simulink model "EvReferenceApplication"  (R2018a)
settings: Solver=ode23tb  StartTime=0  StopTime=ttime  RelTol=1e-3  EnableMultiTasking=on
InitFcn:
  | open_system('EvReferenceApplication/Visualization/Performance and FE Scope');
undefined symbols (not defined in the file): const, const1, const2, Grade
libraries: autolibshared x5
settings Model: ModifiedByFormat=The MathWorks, Inc.  SimulationMode=accelerator  PauseTimes=23.46  Creator=The MathWorks, Inc.  LastModifiedBy=The MathWorks, Inc.
settings SolverCC: DecoupledContinuousIntegration=on
settings DataIOCC: DSMLogging=off
settings DebuggingCC: AlgebraicLoopMsg=none  UnderspecifiedInitializationDetection=Classic  MergeDetectMultiDrivingBlocksExec=none  ModelReferenceExtraNoncontSigs=none
settings ModelReferenceCC: UpdateModelReferenceTargets=IfOutOfDate  EnableParallelModelReferenceBuilds=on  ModelReferenceMinAlgLoopOccurrences=on  PropagateSignalLabelsOutOfModel=off
settings CodeAppCC: StateflowObjectComments=on
settings GRTTargetCC: TargetLangStandard=C89/C90 (ANSI)
settings ConfigComp: CovMetricSettings=dsw  CovHtmlReporting=on  CovSaveCumulativeToWorkspaceVar=on  CovSaveSingleToWorkspaceVar=on  CovShowResultsExplorer=off  CovExternalEMLEnable=off

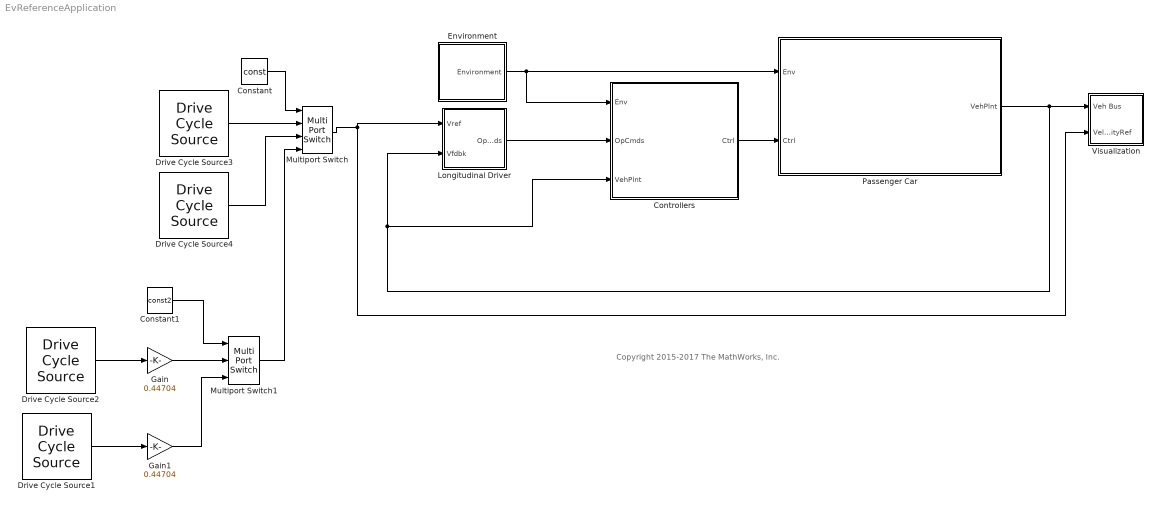
== system EvReferenceApplication ==
  note: Copyright 2015-2017 The MathWorks, Inc.
  Constant : Constant  Value=const
  Constant1 : Constant  Value=const2
  Controllers : Subsystem
      mask Display: image('SystemControllers.png','center')
  Drive Cycle Source1 : autolibshared/Drive Cycle Source  cycleVar=.mat, .xls, .xlsx or .txt file  fileVar=C:\Users\Umar\Software\Matlab\Projects\EV_4\EV\hwfe_1Hz.csv  tfinal="775  seconds"  cycleRepeat=off  outAccPort=off  outGearPort=off  gearList=No gear data  t_wot1=5  xdot_woto=50  xdot_wot1=300  t_wot2=300  xdot_wot2=50  t_wotend=310  srcUnit=mph  outUnit=mph  srcAccUnit=m/s/s  outAccUnit=m/s^2  dt=0  aMode=1
      settings: SourceProductName=Powertrain Blockset  SourceProductBaseCode=PW
  Drive Cycle Source2 : autolibshared/Drive Cycle Source  cycleVar=.mat, .xls, .xlsx or .txt file  fileVar=C:\Users\Umar\Software\Matlab\Projects\EV_4\EV\FTPMC1B.csv  tfinal="1874  seconds"  cycleRepeat=off  outAccPort=off  outGearPort=off  gearList=No gear data  t_wot1=5  xdot_woto=50  xdot_wot1=300  t_wot2=300  xdot_wot2=50  t_wotend=310  srcUnit=mph  outUnit=mph  srcAccUnit=m/s/s  outAccUnit=m/s^2  dt=0  aMode=1
      settings: SourceProductName=Powertrain Blockset  SourceProductBaseCode=PW
  Drive Cycle Source3 : autolibshared/Drive Cycle Source  cycleVar=FTP75  fileVar=L:\Bauto\matlab\test\toolbox\shared\autoblks\scenario\adac.txt  tfinal="2474  seconds"  cycleRepeat=off  outAccPort=off  outGearPort=off  gearList=No gear data  t_wot1=5  xdot_woto=0  xdot_wot1=30  t_wot2=20  xdot_wot2=0  t_wotend=30  srcUnit=m/s  outUnit=m/s  srcAccUnit=m/s/s  outAccUnit=m/s^2  dt=0  aMode=1
      settings: SourceProductName=Powertrain Blockset  SourceProductBaseCode=PW
  Drive Cycle Source4 : autolibshared/Drive Cycle Source  cycleVar=Wide Open Throttle (WOT)  fileVar=L:\Bauto\matlab\test\toolbox\shared\autoblks\scenario\adac.txt  tfinal="310  seconds"  cycleRepeat=off  outAccPort=off  outGearPort=off  gearList=No gear data  t_wot1=5  xdot_woto=0  xdot_wot1=300  t_wot2=300  xdot_wot2=0  t_wotend=310  srcUnit=m/s  outUnit=m/s  srcAccUnit=m/s/s  outAccUnit=m/s^2  dt=0  aMode=1
      settings: SourceProductName=Powertrain Blockset  SourceProductBaseCode=PW
  Environment : Subsystem
      mask Display: disp('Environment')
  Gain : Gain  Gain=0.44704
  Gain1 : Gain  Gain=0.44704
  Longitudinal Driver : Subsystem
      mask Display: image('LongitudinalDriver.png', 'center')
  Multiport Switch : MultiPortSwitch
  Multiport Switch1 : MultiPortSwitch  Inputs=2
  Passenger Car : Subsystem
      mask Display: image('PassengerVehicle.png','center')
  Visualization : Subsystem
      mask Display: disp('Visualization')
  wires:
  Longitudinal Driver/1(OpCmds) -> Controllers/2(OpCmds)
  Environment/1(Environment) -> Controllers/1(Env), Passenger Car/1(Env)
  Controllers/1(Ctrl) -> Passenger Car/2(Ctrl)
  Passenger Car/1(VehPlnt) -> Controllers/3(VehPlnt), Longitudinal Driver/2(Vfdbk), Visualization/1(Veh Bus)
  Multiport Switch/1 -> Longitudinal Driver/1(Vref), Visualization/2(VelocityRef)
  Drive Cycle Source3/1 -> Multiport Switch/2
  Constant/1 -> Multiport Switch/1
  Drive Cycle Source4/1 -> Multiport Switch/3
  Drive Cycle Source2/1 -> Gain/1
  Drive Cycle Source1/1 -> Gain1/1
  Multiport Switch1/1 -> Multiport Switch/4
  Constant1/1 -> Multiport Switch1/1
  Gain/1 -> Multiport Switch1/2
  Gain1/1 -> Multiport Switch1/3

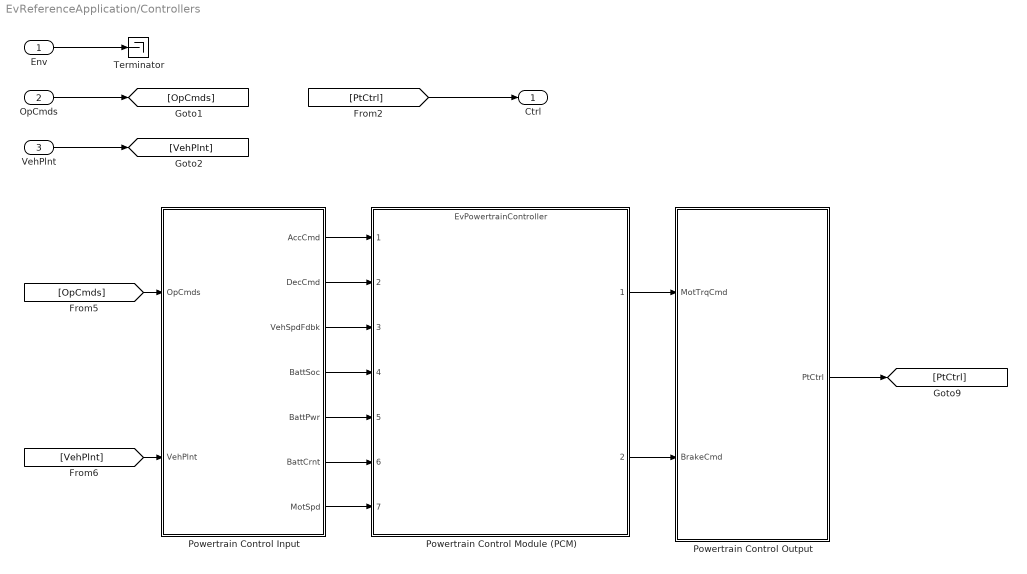
== system EvReferenceApplication/Controllers ==
  Env : Inport
  OpCmds : Inport  Port=2
  VehPlnt : Inport  Port=3
  Powertrain Control Input : Subsystem
  Powertrain Control Module (PCM) : ModelReference  ModelNameDialog=EvPowertrainController  ModelReferenceVersion=1.403
  Powertrain Control Output : Subsystem
  Terminator : Terminator
  Ctrl : Outport
  wires:
  [PtCtrl] -> Ctrl/1
  Env/1 -> Terminator/1
  [OpCmds] -> Powertrain Control Input/1(OpCmds)
  Powertrain Control Output/1(PtCtrl) -> [PtCtrl]
  [VehPlnt] -> Powertrain Control Input/2(VehPlnt)
  VehPlnt/1 -> [VehPlnt]
  OpCmds/1 -> [OpCmds]
  Powertrain Control Input/4(BattSoc) -> Powertrain Control Module (PCM)/4
  Powertrain Control Input/3(VehSpdFdbk) -> Powertrain Control Module (PCM)/3
  Powertrain Control Input/2(DecCmd) -> Powertrain Control Module (PCM)/2
  Powertrain Control Input/1(AccCmd) -> Powertrain Control Module (PCM)/1
  Powertrain Control Input/5(BattPwr) -> Powertrain Control Module (PCM)/5
  Powertrain Control Input/6(BattCrnt) -> Powertrain Control Module (PCM)/6
  Powertrain Control Input/7(MotSpd) -> Powertrain Control Module (PCM)/7
  Powertrain Control Module (PCM)/1 -> Powertrain Control Output/1(MotTrqCmd)
  Powertrain Control Module (PCM)/2 -> Powertrain Control Output/2(BrakeCmd)

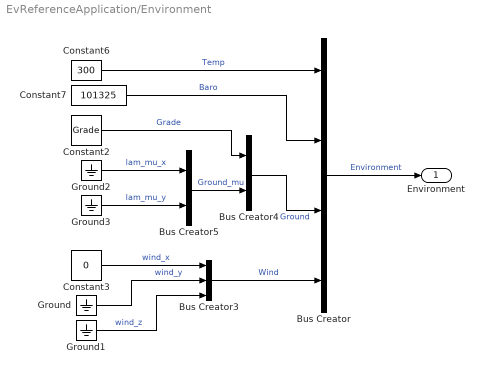
== system EvReferenceApplication/Environment ==
  Bus Creator : BusCreator  Inputs=4
  Bus Creator3 : BusCreator  Inputs=3
  Bus Creator4 : BusCreator  Inputs=2
  Bus Creator5 : BusCreator  Inputs=2
  Constant2 : Constant  Value=Grade
  Constant3 : Constant  Value=0
  Constant6 : Constant  Value=300
  Constant7 : Constant  Value=101325
  Ground{,1..3} (4 alike) : Ground
  Environment : Outport
  wires:
  Ground2/1 -> Bus Creator5/1  "lam_mu_x"
  Ground3/1 -> Bus Creator5/2  "lam_mu_y"
  Bus Creator5/1 -> Bus Creator4/2  "Ground_mu"
  Bus Creator4/1 -> Bus Creator/3  "Ground"
  Bus Creator3/1 -> Bus Creator/4  "Wind"
  Constant3/1 -> Bus Creator3/1  "wind_x"
  Ground/1 -> Bus Creator3/2  "wind_y"
  Ground1/1 -> Bus Creator3/3  "wind_z"
  Constant6/1 -> Bus Creator/1  "Temp"
  Constant2/1 -> Bus Creator4/1  "Grade"
  Bus Creator/1 -> Environment/1  "Environment"
  Constant7/1 -> Bus Creator/2  "Baro"

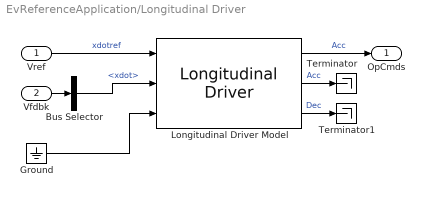
== system EvReferenceApplication/Longitudinal Driver ==
  Vref : Inport
  Vfdbk : Inport  Port=2
  Bus Selector : BusSelector  OutputSignals=Veh.xdot
  Ground : Ground
  Longitudinal Driver Model : autolibshared/Longitudinal Driver  aMode=1  vnom=5  Kp=1.5  Ki=1.5  Kaw=1  Kff=.1  Kg=0  tauerr=0.01
      settings: SourceProductName=Powertrain Blockset  SourceProductBaseCode=PW
  Terminator : Terminator
  Terminator1 : Terminator
  OpCmds : Outport
  wires:
  Bus Selector/1 -> Longitudinal Driver Model/2  "<xdot>"
  Vref/1 -> Longitudinal Driver Model/1  "xdotref"
  Vfdbk/1 -> Bus Selector/1
  Longitudinal Driver Model/1 -> OpCmds/1  "Acc"
  Longitudinal Driver Model/2 -> Terminator/1  "Acc"
  Longitudinal Driver Model/3 -> Terminator1/1  "Dec"
  Ground/1 -> Longitudinal Driver Model/3

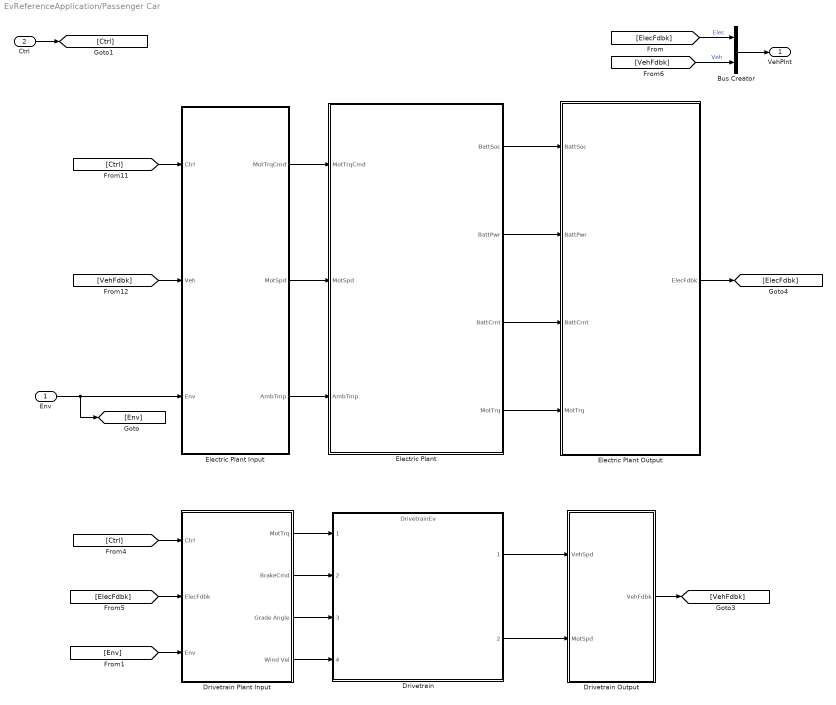
== system EvReferenceApplication/Passenger Car ==
  Env : Inport
  Ctrl : Inport  Port=2
  Bus Creator : BusCreator  Inputs=2
  Drivetrain : ModelReference  ModelNameDialog=DrivetrainEv.slx  SimulationMode=Normal  ModelReferenceVersion=1.431
  Drivetrain Output : Subsystem
  Drivetrain Plant Input : Subsystem
  Electric Plant : Subsystem
  Electric Plant Input : Subsystem
  Electric Plant Output : Subsystem
  VehPlnt : Outport
  wires:
  Ctrl/1 -> [Ctrl]
  Env/1 -> [Env], Electric Plant Input/3(Env)
  [Ctrl] -> Drivetrain Plant Input/1(Ctrl)
  Bus Creator/1 -> VehPlnt/1
  [VehFdbk] -> Bus Creator/2  "Veh"
  Drivetrain Output/1(VehFdbk) -> [VehFdbk]
  Electric Plant Output/1(ElecFdbk) -> [ElecFdbk]
  [ElecFdbk] -> Bus Creator/1  "Elec"
  [Ctrl] -> Electric Plant Input/1(Ctrl)
  [ElecFdbk] -> Drivetrain Plant Input/2(ElecFdbk)
  [VehFdbk] -> Electric Plant Input/2(Veh)
  Drivetrain Plant Input/2(BrakeCmd) -> Drivetrain/2
  Drivetrain Plant Input/1(MotTrq) -> Drivetrain/1
  Drivetrain/2 -> Drivetrain Output/2(MotSpd)
  Drivetrain/1 -> Drivetrain Output/1(VehSpd)
  Electric Plant Input/1(MotTrqCmd) -> Electric Plant/1(MotTrqCmd)
  Electric Plant Input/2(MotSpd) -> Electric Plant/2(MotSpd)
  Electric Plant/1(BattSoc) -> Electric Plant Output/1(BattSoc)
  Electric Plant/2(BattPwr) -> Electric Plant Output/2(BattPwr)
  Electric Plant/3(BattCrnt) -> Electric Plant Output/3(BattCrnt)
  Electric Plant/4(MotTrq) -> Electric Plant Output/4(MotTrq)
  Electric Plant Input/3(AmbTmp) -> Electric Plant/3(AmbTmp)
  [Env] -> Drivetrain Plant Input/3(Env)
  Drivetrain Plant Input/3(Grade Angle) -> Drivetrain/3
  Drivetrain Plant Input/4(Wind Vel) -> Drivetrain/4

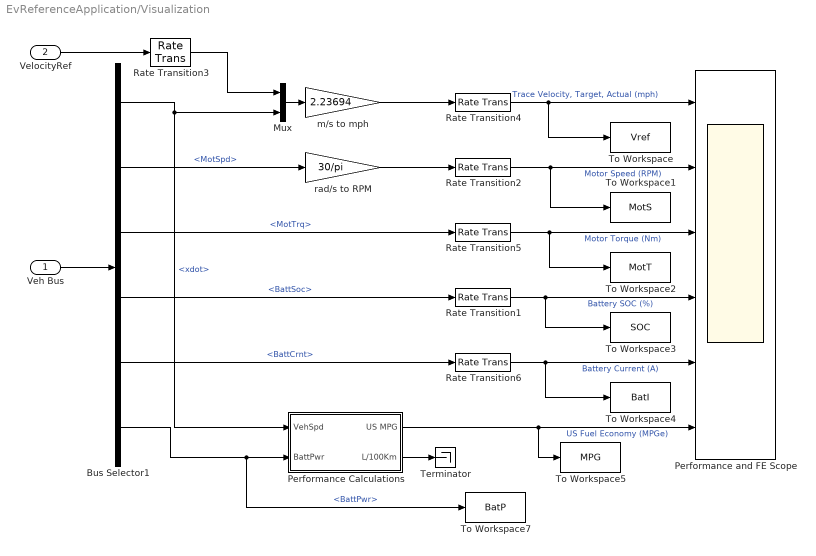
== system EvReferenceApplication/Visualization ==
  Veh Bus : Inport
  VelocityRef : Inport  Port=2
  Bus Selector1 : BusSelector  OutputSignals=Veh.xdot,Veh.MotSpd,Elec.MotTrq,Elec.BattSoc,Elec.BattCrnt,Elec.BattPwr
  Mux : Mux  Inputs=2
  Performance Calculations : Subsystem
  Performance and FE Scope : Scope  NumInputPorts=6
  Rate Transition{1..6} (6 alike) : RateTransition
  Terminator : Terminator
  To Workspace : ToWorkspace  VariableName=Vref  SaveFormat=Timeseries  SampleTime=1
  To Workspace1 : ToWorkspace  VariableName=MotS  SaveFormat=Timeseries  SampleTime=1
  To Workspace2 : ToWorkspace  VariableName=MotT  SaveFormat=Timeseries  SampleTime=1
  To Workspace3 : ToWorkspace  VariableName=SOC  SaveFormat=Timeseries  SampleTime=1
  To Workspace4 : ToWorkspace  VariableName=BatI  SaveFormat=Timeseries  SampleTime=1
  To Workspace5 : ToWorkspace  VariableName=MPG  SaveFormat=Timeseries  SampleTime=1
  To Workspace7 : ToWorkspace  VariableName=BatP  SaveFormat=Timeseries  SampleTime=1
  m/s to mph : Gain  Gain=2.23694
  rad/s to RPM : Gain  Gain=30/pi
  wires:
  Veh Bus/1 -> Bus Selector1/1
  Bus Selector1/1 -> Performance Calculations/1(VehSpd), Mux/2  "<xdot>"
  Mux/1 -> m/s to mph/1
  Performance Calculations/1(US MPG) -> To Workspace5/1, Performance and FE Scope/6  "US Fuel Economy (MPGe)"
  Performance Calculations/2(L/100Km) -> Terminator/1
  m/s to mph/1 -> Rate Transition4/1
  VelocityRef/1 -> Rate Transition3/1
  Bus Selector1/4 -> Rate Transition1/1  "<BattSoc>"
  Rate Transition3/1 -> Mux/1
  Rate Transition1/1 -> To Workspace3/1, Performance and FE Scope/4  "Battery SOC (%)"
  Rate Transition2/1 -> To Workspace1/1, Performance and FE Scope/2  "Motor Speed (RPM)"
  Rate Transition4/1 -> To Workspace/1, Performance and FE Scope/1  "Trace Velocity, Target, Actual (mph)"
  Bus Selector1/2 -> rad/s to RPM/1  "<MotSpd>"
  Bus Selector1/6 -> To Workspace7/1, Performance Calculations/2(BattPwr)  "<BattPwr>"
  rad/s to RPM/1 -> Rate Transition2/1
  Bus Selector1/3 -> Rate Transition5/1  "<MotTrq>"
  Rate Transition5/1 -> To Workspace2/1, Performance and FE Scope/3  "Motor Torque (Nm)"
  Rate Transition6/1 -> To Workspace4/1, Performance and FE Scope/5  "Battery Current (A)"
  Bus Selector1/5 -> Rate Transition6/1  "<BattCrnt>"

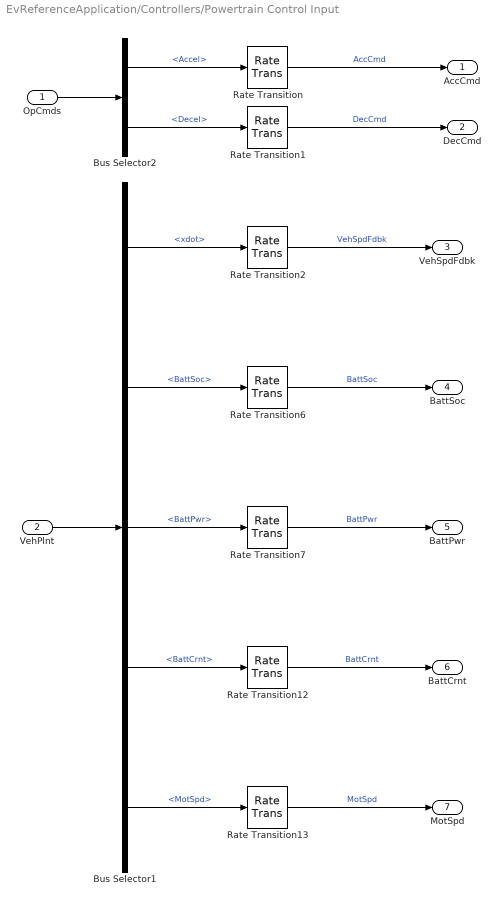
== system EvReferenceApplication/Controllers/Powertrain Control Input ==
  OpCmds : Inport
  VehPlnt : Inport  Port=2
  Bus Selector1 : BusSelector  OutputSignals=Veh.xdot,Elec.BattSoc,Elec.BattPwr,Elec.BattCrnt,Veh.MotSpd
  Bus Selector2 : BusSelector  OutputSignals=Accel,Decel
  Rate Transition{,1..2,6..7,12..13} (7 alike) : RateTransition  Deterministic=off
  AccCmd : Outport
  DecCmd : Outport  Port=2
  VehSpdFdbk : Outport  Port=3
  BattSoc : Outport  Port=4
  BattPwr : Outport  Port=5
  BattCrnt : Outport  Port=6
  MotSpd : Outport  Port=7
  wires:
  Bus Selector2/1 -> Rate Transition/1  "<Accel>"
  Rate Transition/1 -> AccCmd/1  "AccCmd"
  OpCmds/1 -> Bus Selector2/1
  Bus Selector2/2 -> Rate Transition1/1  "<Decel>"
  Rate Transition1/1 -> DecCmd/1  "DecCmd"
  Rate Transition2/1 -> VehSpdFdbk/1  "VehSpdFdbk"
  VehPlnt/1 -> Bus Selector1/1
  Rate Transition6/1 -> BattSoc/1  "BattSoc"
  Rate Transition7/1 -> BattPwr/1  "BattPwr"
  Rate Transition12/1 -> BattCrnt/1  "BattCrnt"
  Bus Selector1/1 -> Rate Transition2/1  "<xdot>"
  Bus Selector1/2 -> Rate Transition6/1  "<BattSoc>"
  Bus Selector1/3 -> Rate Transition7/1  "<BattPwr>"
  Bus Selector1/4 -> Rate Transition12/1  "<BattCrnt>"
  Rate Transition13/1 -> MotSpd/1  "MotSpd"
  Bus Selector1/5 -> Rate Transition13/1  "<MotSpd>"

== system EvReferenceApplication/Controllers/Powertrain Control Output ==
  MotTrqCmd : Inport
  BrakeCmd : Inport  Port=2
  Bus Creator : BusCreator  Inputs=2
  Rate Transition1 : RateTransition  Deterministic=off
  Rate Transition5 : RateTransition  Deterministic=off
  PtCtrl : Outport
  wires:
  Rate Transition1/1 -> Bus Creator/2  "BrakeCmd"
  BrakeCmd/1 -> Rate Transition1/1
  Bus Creator/1 -> PtCtrl/1  "PtCtrl"
  Rate Transition5/1 -> Bus Creator/1  "MotTrqCmd"
  MotTrqCmd/1 -> Rate Transition5/1

== system EvReferenceApplication/Passenger Car/Drivetrain Output ==
  VehSpd : Inport
  MotSpd : Inport  Port=2
  Bus Creator1 : BusCreator  Inputs=2
  VehFdbk : Outport
  wires:
  Bus Creator1/1 -> VehFdbk/1  "VehFdbk"
  VehSpd/1 -> Bus Creator1/1
  MotSpd/1 -> Bus Creator1/2  "MotSpd"

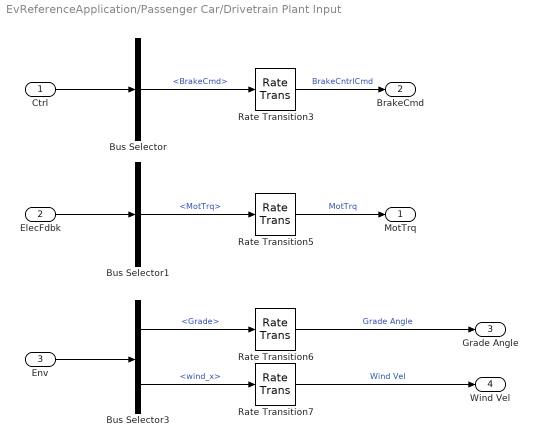
== system EvReferenceApplication/Passenger Car/Drivetrain Plant Input ==
  Ctrl : Inport
  ElecFdbk : Inport  Port=2
  Env : Inport  Port=3
  Bus Selector : BusSelector  OutputSignals=BrakeCmd
  Bus Selector1 : BusSelector  OutputSignals=MotTrq
  Bus Selector3 : BusSelector  OutputSignals=Ground.Grade,Wind.wind_x
  Rate Transition{3,5..7} (4 alike) : RateTransition  Deterministic=off
  MotTrq : Outport
  BrakeCmd : Outport  Port=2
  Grade Angle : Outport  Port=3
  Wind Vel : Outport  Port=4
  wires:
  Ctrl/1 -> Bus Selector/1
  Bus Selector/1 -> Rate Transition3/1  "<BrakeCmd>"
  Rate Transition3/1 -> BrakeCmd/1  "BrakeCntrlCmd"
  ElecFdbk/1 -> Bus Selector1/1
  Rate Transition5/1 -> MotTrq/1  "MotTrq"
  Bus Selector1/1 -> Rate Transition5/1  "<MotTrq>"
  Env/1 -> Bus Selector3/1
  Rate Transition6/1 -> Grade Angle/1  "Grade Angle"
  Rate Transition7/1 -> Wind Vel/1  "Wind Vel"
  Bus Selector3/1 -> Rate Transition6/1  "<Grade>"
  Bus Selector3/2 -> Rate Transition7/1  "<wind_x>"

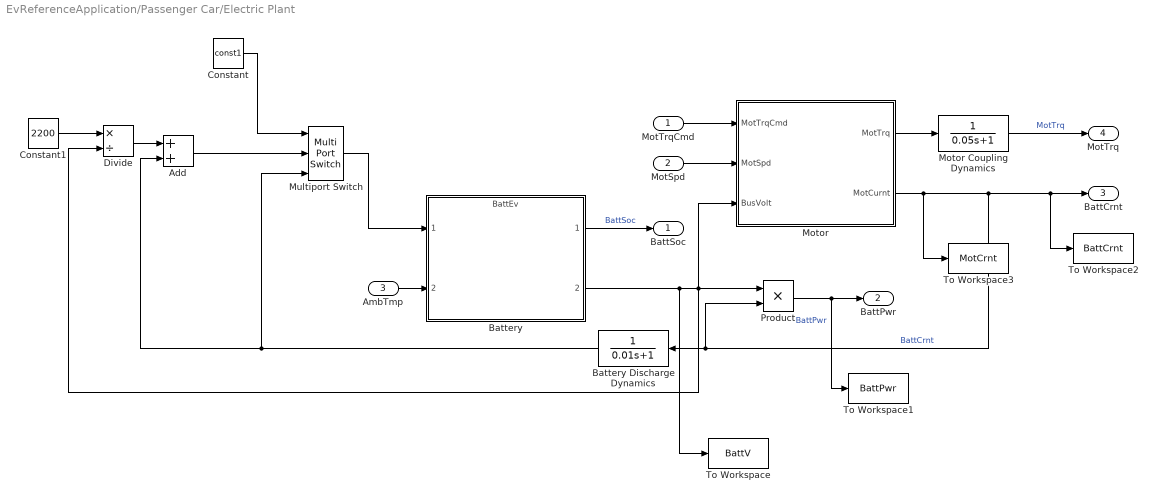
== system EvReferenceApplication/Passenger Car/Electric Plant ==
  MotTrqCmd : Inport
  MotSpd : Inport  Port=2
  AmbTmp : Inport  Port=3
  Add : Sum
  Battery : ModelReference  ModelNameDialog=BattEv.slx  SimulationMode=Normal  ModelReferenceVersion=1.369
  Battery Discharge Dynamics : TransferFcn  Denominator=[0.01 1]
  Constant : Constant  Value=const1
  Constant1 : Constant  Value=2200
  Divide : Product  Inputs=*/
  Motor : Subsystem  Variant=on  OverrideUsingVariant=MotGenEvMapped
  Motor Coupling Dynamics : TransferFcn  Denominator=[0.05 1]
  Multiport Switch : MultiPortSwitch  Inputs=2
  Product : Product
  To Workspace : ToWorkspace  VariableName=BattV  SaveFormat=Timeseries  SampleTime=-1
  To Workspace1 : ToWorkspace  VariableName=BattPwr  SaveFormat=Timeseries  SampleTime=-1
  To Workspace2 : ToWorkspace  VariableName=BattCrnt  SaveFormat=Timeseries  SampleTime=-1
  To Workspace3 : ToWorkspace  VariableName=MotCrnt  SaveFormat=Timeseries  SampleTime=-1
  BattSoc : Outport
  BattPwr : Outport  Port=2
  BattCrnt : Outport  Port=3
  MotTrq : Outport  Port=4
  wires:
  MotTrqCmd/1 -> Motor/1(MotTrqCmd)
  MotSpd/1 -> Motor/2(MotSpd)
  AmbTmp/1 -> Battery/2
  Motor/1(MotTrq) -> Motor Coupling Dynamics/1
  Battery/1 -> BattSoc/1  "BattSoc"
  Battery/2 -> To Workspace/1, Divide/2, Motor/3(BusVolt), Product/1
  Product/1 -> To Workspace1/1, BattPwr/1  "BattPwr"
  Motor/2(MotCurnt) -> Battery Discharge Dynamics/1, Product/2, To Workspace2/1, BattCrnt/1, To Workspace3/1  "BattCrnt"
  Battery Discharge Dynamics/1 -> Multiport Switch/3, Add/2
  Motor Coupling Dynamics/1 -> MotTrq/1  "MotTrq"
  Constant/1 -> Multiport Switch/1
  Constant1/1 -> Divide/1
  Divide/1 -> Add/1
  Add/1 -> Multiport Switch/2
  Multiport Switch/1 -> Battery/1

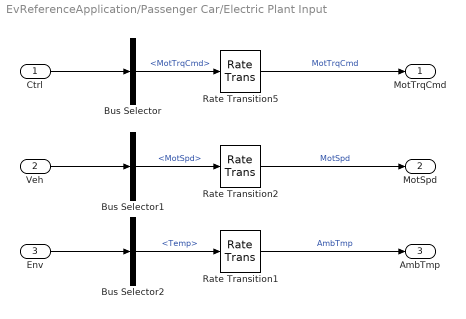
== system EvReferenceApplication/Passenger Car/Electric Plant Input ==
  Ctrl : Inport
  Veh : Inport  Port=2
  Env : Inport  Port=3
  Bus Selector : BusSelector  OutputSignals=MotTrqCmd
  Bus Selector1 : BusSelector  OutputSignals=MotSpd
  Bus Selector2 : BusSelector  OutputSignals=Temp
  Rate Transition1 : RateTransition  Deterministic=off
  Rate Transition2 : RateTransition  Deterministic=off
  Rate Transition5 : RateTransition  Deterministic=off
  MotTrqCmd : Outport
  MotSpd : Outport  Port=2
  AmbTmp : Outport  Port=3
  wires:
  Rate Transition5/1 -> MotTrqCmd/1  "MotTrqCmd"
  Ctrl/1 -> Bus Selector/1
  Bus Selector/1 -> Rate Transition5/1  "<MotTrqCmd>"
  Veh/1 -> Bus Selector1/1
  Rate Transition2/1 -> MotSpd/1  "MotSpd"
  Bus Selector1/1 -> Rate Transition2/1  "<MotSpd>"
  Env/1 -> Bus Selector2/1
  Rate Transition1/1 -> AmbTmp/1  "AmbTmp"
  Bus Selector2/1 -> Rate Transition1/1  "<Temp>"

== system EvReferenceApplication/Passenger Car/Electric Plant Output ==
  BattSoc : Inport
  BattPwr : Inport  Port=2
  BattCrnt : Inport  Port=3
  MotTrq : Inport  Port=4
  Bus Creator1 : BusCreator  Inputs=4
  ElecFdbk : Outport
  wires:
  Bus Creator1/1 -> ElecFdbk/1  "ElecFdbk"
  BattPwr/1 -> Bus Creator1/2
  BattSoc/1 -> Bus Creator1/1
  BattCrnt/1 -> Bus Creator1/3
  MotTrq/1 -> Bus Creator1/4

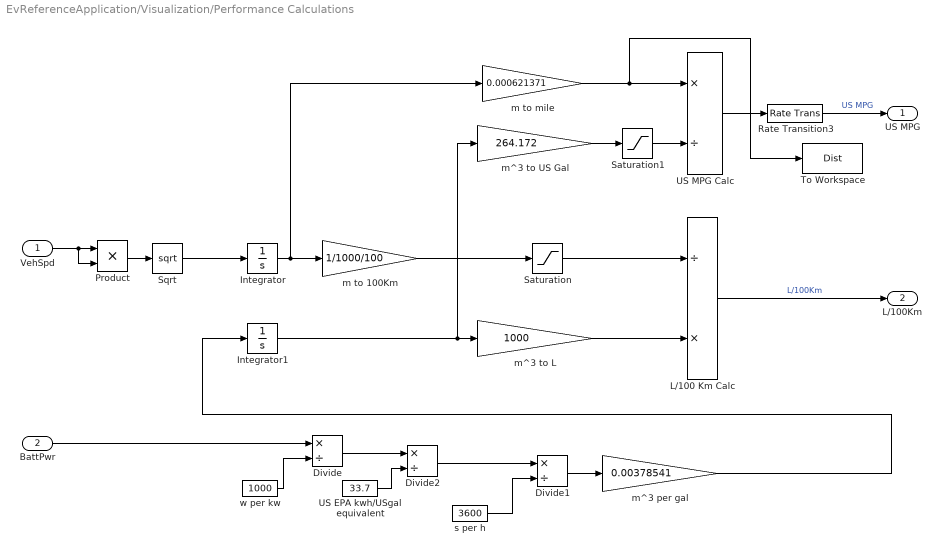
== system EvReferenceApplication/Visualization/Performance Calculations ==
  VehSpd : Inport
  BattPwr : Inport  Port=2
  Divide : Product  Inputs=*/
  Divide1 : Product  Inputs=*/
  Divide2 : Product  Inputs=*/
  Integrator : Integrator
  Integrator1 : Integrator
  L/100 Km Calc : Product  Inputs=/*
  Product : Product
  Rate Transition3 : RateTransition
  Saturation : Saturate  UpperLimit=Inf  LowerLimit=0.1
  Saturation1 : Saturate  UpperLimit=Inf  LowerLimit=1e-3
  Sqrt : Sqrt  SaturateOnIntegerOverflow=on
  To Workspace : ToWorkspace  VariableName=Dist  SaveFormat=Timeseries  SampleTime=1
  US EPA kwh/USgal equivalent : Constant  Value=33.7
  US MPG Calc : Product  Inputs=*/
  m to 100Km : Gain  Gain=1/1000/100
  m to mile : Gain  Gain=0.000621371
  m^3 per gal : Gain  Gain=0.00378541
  m^3 to L : Gain  Gain=1000
  m^3 to US Gal : Gain  Gain=264.172
  s per h : Constant  Value=3600
  w per kw : Constant  Value=1000
  US MPG : Outport
  L/100Km : Outport  Port=2
  wires:
  m^3 to US Gal/1 -> Saturation1/1
  m^3 to L/1 -> L/100 Km Calc/2
  Integrator/1 -> m to mile/1, m to 100Km/1
  m to mile/1 -> To Workspace/1, US MPG Calc/1
  Integrator1/1 -> m^3 to US Gal/1, m^3 to L/1
  Saturation/1 -> L/100 Km Calc/1
  m to 100Km/1 -> Saturation/1
  L/100 Km Calc/1 -> L/100Km/1  "L/100Km"
  US MPG Calc/1 -> Rate Transition3/1
  Saturation1/1 -> US MPG Calc/2
  Rate Transition3/1 -> US MPG/1  "US MPG"
  w per kw/1 -> Divide/2
  Divide/1 -> Divide2/1
  Divide2/1 -> Divide1/1
  s per h/1 -> Divide1/2
  Divide1/1 -> m^3 per gal/1
  m^3 per gal/1 -> Integrator1/1
  US EPA kwh/USgal equivalent/1 -> Divide2/2
  BattPwr/1 -> Divide/1
  Sqrt/1 -> Integrator/1
  Product/1 -> Sqrt/1
  VehSpd/1 -> Product/2, Product/1

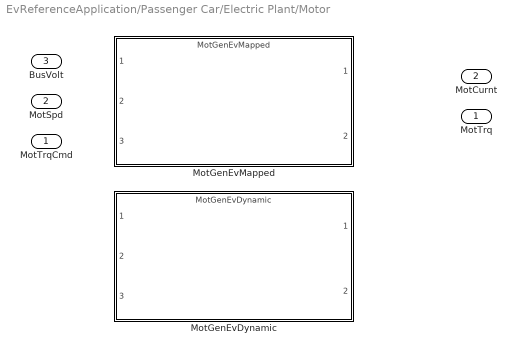
== system EvReferenceApplication/Passenger Car/Electric Plant/Motor ==
  MotTrqCmd : Inport
  MotSpd : Inport  Port=2
  BusVolt : Inport  Port=3
  MotGenEvDynamic : ModelReference  ModelNameDialog=MotGenEvDynamic.slx  SimulationMode=Normal  VariantControl=MotGenEvDynamic  ModelReferenceVersion=1.346
  MotGenEvMapped : ModelReference  ModelNameDialog=MotGenEvMapped.slx  SimulationMode=Normal  VariantControl=MotGenEvMapped  ModelReferenceVersion=1.351
  MotTrq : Outport
  MotCurnt : Outport  Port=2
